simulink model "relative_movement_and_rotation"  (R2019b)
settings: Solver=VariableStepAuto  StartTime=0.0  StopTime=10.0  RelTol=1e-3
libraries: blocklib x3, vrlib x2
settings Model: Creator=imanol  LastModifiedBy=imanol

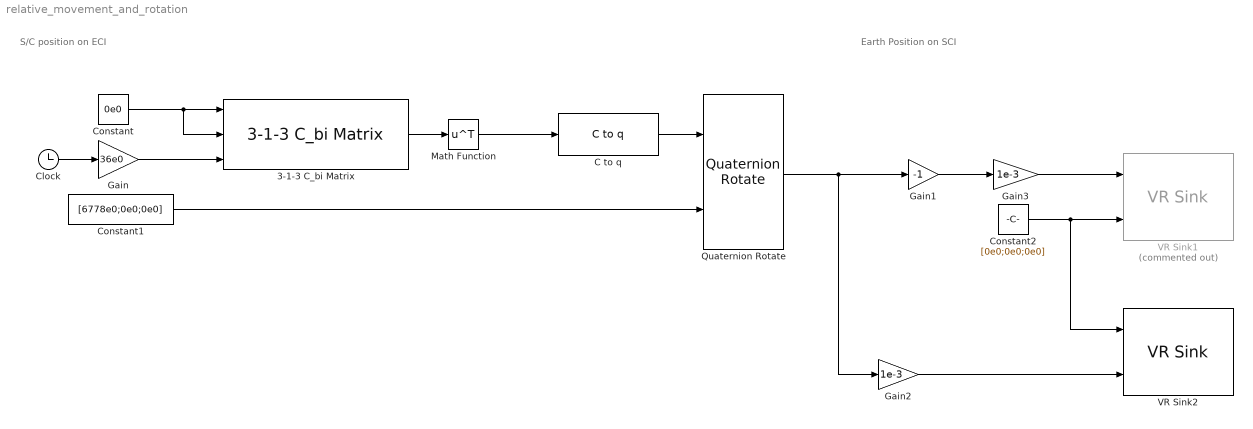
== system relative_movement_and_rotation ==
  note: Earth Position on SCI
  note: S/C position on ECI
  3-1-3 C_bi Matrix : blocklib/3-1-3 C_bi Matrix  Tag=|  SystemSampleTime=-1  Latency=0  AutoFrameSizeCalculation=off
      | text(.05,.5,'{\itEquation:}  \Sigma \alpha^2 + 
      | \beta^2 \rightarrow \infty, \Pi, \phi_3 = {\bfcool}', 
      | 'hor','left','texmode','on')
      settings: SourceProductName=Custom Library
  C to q : blocklib/C to q  SystemSampleTime=-1  Latency=0  AutoFrameSizeCalculation=off
      settings: SourceProductName=Custom Library
  Clock : Clock
  Constant : Constant  Value=0e0
  Constant1 : Constant  Value=[6778e0;0e0;0e0]
  Constant2 : Constant  Value=[0e0;0e0;0e0]
  Gain : Gain  Gain=36e0
  Gain1 : Gain  Gain=-1
  Gain2 : Gain  Gain=1e-3
  Gain3 : Gain  Gain=1e-3
  Math Function : Math  Operator=transpose  SignedPower=off  SaturateOnIntegerOverflow=on
  Quaternion Rotate : blocklib/Quaternion Rotate  SystemSampleTime=-1  Latency=0  AutoFrameSizeCalculation=off
      settings: SourceProductName=Custom Library
  VR Sink1 : vrlib/VR Sink  Commented=on  InstantiateOnLoad=on  SampleTime=0.1  ViewEnable=on  RemoteChange=off  RemoteView=off  FieldsWritten=Earth.translation.3.1.1.double#S/C.translation.3.1.1.double  WorldFileName=relative_movement.wrl  AutoView=off  VideoDimensions=[]  AllowVariableSize=off
      settings: SourceProductName=Simulink
  VR Sink2 : vrlib/VR Sink  InstantiateOnLoad=on  SampleTime=0.1  ViewEnable=on  RemoteChange=off  RemoteView=off  FieldsWritten=Earth.translation.3.1.1.double#S/C.translation.3.1.1.double  WorldFileName=relative_movement.wrl  AutoView=off  VideoDimensions=[]  AllowVariableSize=off
      settings: SourceProductName=Simulink
  wires:
  Quaternion Rotate/1 -> Gain2/1, Gain1/1
  3-1-3 C_bi Matrix/1 -> Math Function/1
  Gain/1 -> 3-1-3 C_bi Matrix/3
  Constant/1 -> 3-1-3 C_bi Matrix/2, 3-1-3 C_bi Matrix/1
  Math Function/1 -> C to q/1
  C to q/1 -> Quaternion Rotate/1
  Constant1/1 -> Quaternion Rotate/2
  Clock/1 -> Gain/1
  Gain2/1 -> VR Sink2/2
  Constant2/1 -> VR Sink2/1, VR Sink1/2
  Gain1/1 -> Gain3/1
  Gain3/1 -> VR Sink1/1
